simulink model "Mechanical_Accelerometer"  (R2024a)
settings: Solver=VariableStepAuto  StartTime=0.0  StopTime=50  MaxStep=0.01  RelTol=1e-3
model workspace (MAT data in the model file):
  M = 10
  Ms = 100
  b = 12
  k = 32
settings Model: Creator=91839
settings SolverCC: AlgebraicLoopSolver=TrustRegion
settings DataIOCC: ExternalInput=data  LoadExternalInput=on  SaveFormat=Array  DSMLogging=off  ReturnWorkspaceOutputs=off
settings DebuggingCC: UnconnectedInputMsg=warning  UnconnectedOutputMsg=warning  UnconnectedLineMsg=warning
settings ModelReferenceCC: EnableRefExpFcnMdlSchedulingChecks=on
settings SFSimCC: CustomCodeUndefinedFunction=UseInterfaceOnly
settings RTWCC: GPUComputeCapability=3.5

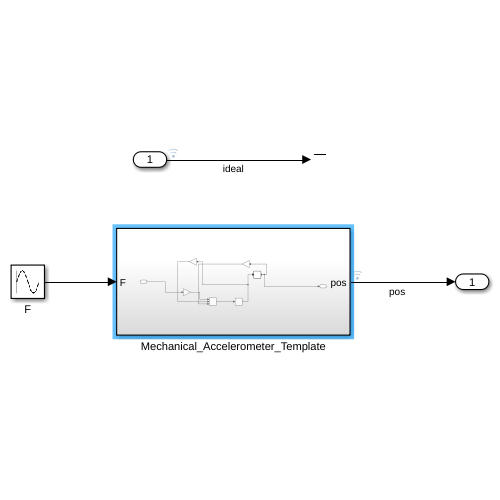
[thumbnail: Simulink's stored preview of the top-level diagram]
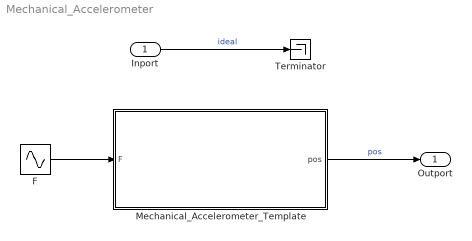
== system Mechanical_Accelerometer ==
  Inport : Inport
  F : Sin  Amplitude=3  SampleTime=0
  Mechanical_Accelerometer_Template : Subsystem
  Terminator : Terminator
  Outport : Outport
  wires:
  Inport/1 -> Terminator/1  "ideal"
  F/1 -> Mechanical_Accelerometer_Template/1(F)
  Mechanical_Accelerometer_Template/1(pos) -> Outport/1  "pos"

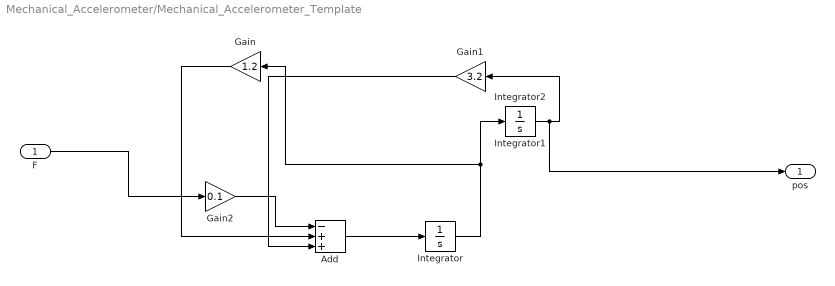
== system Mechanical_Accelerometer/Mechanical_Accelerometer_Template ==
  F : Inport
  Add : Sum  Inputs=-++
  Gain : Gain  Gain=1.2
  Gain1 : Gain  Gain=3.2
  Gain2 : Gain  Gain=0.1
  Integrator : Integrator
  Integrator1 : Integrator
  Integrator2 : Integrator
  pos : Outport
  wires:
  Integrator/1 -> Gain/1, Integrator2/1
  F/1 -> Gain2/1
  Gain2/1 -> Add/1
  Gain/1 -> Add/2
  Gain1/1 -> Add/3
  Add/1 -> Integrator/1
  Integrator2/1 -> pos/1, Gain1/1
